simulink model "ref_model"  (R2025b)
settings: Solver=VariableStepAuto  StartTime=0.0  StopTime=10.0  RelTol=1e-3
settings Model: Creator=JEDIDAH  LastModifiedBy=JEDIDAH

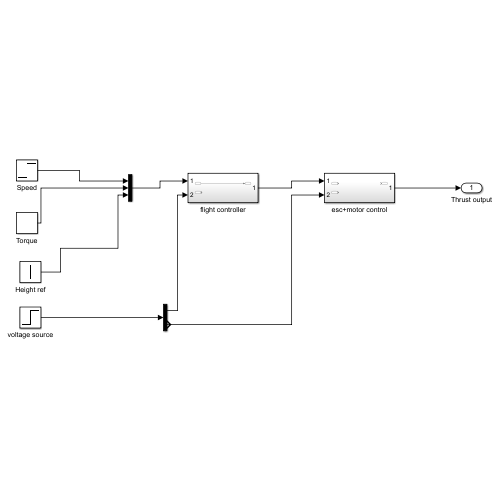
[thumbnail: Simulink's stored preview of the top-level diagram]
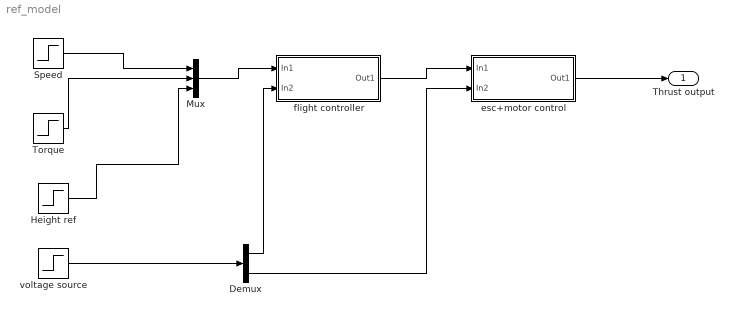
== system ref_model ==
  Demux : Demux  Outputs=2
  Height ref : Step  SampleTime=0
  Mux : Mux  Inputs=3
  Speed : Step  SampleTime=0
  Torque : Step  SampleTime=0
  esc+motor control : Subsystem
  flight controller : Subsystem
  voltage source : Step  SampleTime=0
  Thrust output : Outport
  wires:
  Speed/1 -> Mux/1
  Torque/1 -> Mux/2
  Height ref/1 -> Mux/3
  Mux/1 -> flight controller/1(In1)
  flight controller/1(Out1) -> esc+motor control/1(In1)
  esc+motor control/1(Out1) -> Thrust output/1
  Demux/1 -> flight controller/2(In2)
  voltage source/1 -> Demux/1
  Demux/2 -> esc+motor control/2(In2)

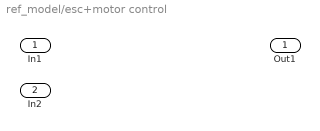
== system ref_model/esc+motor control ==
  In1 : Inport
  In2 : Inport  Port=2
  Out1 : Outport

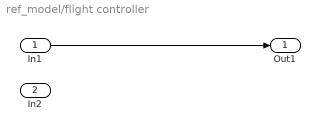
== system ref_model/flight controller ==
  In1 : Inport
  In2 : Inport  Port=2
  Out1 : Outport
  wires:
  In1/1 -> Out1/1
